simulink model "gm_sampleModel1830_1_sub_sub"  (R2023a)
settings: Solver=VariableStepAuto  StartTime=0.0  StopTime=10.0  RelTol=1e-3
libraries: hdlsllib x6, simulink x1
settings Model: Creator=user1  LastModifiedBy=user1
settings OptimizationCC: BlockReduction=off  ConditionallyExecuteInputs=off
settings DebuggingCC: InheritedTsInSrcMsg=none

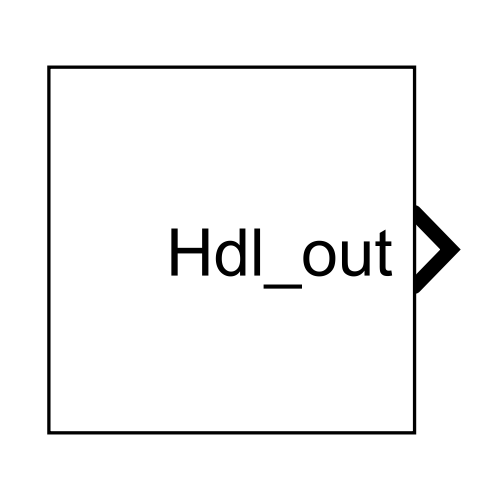
[thumbnail: Simulink's stored preview of the top-level diagram]
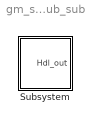
== system gm_sampleModel1830_1_sub_sub ==
  Subsystem : Subsystem

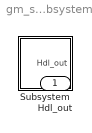
== system gm_sampleModel1830_1_sub_sub/Subsystem ==
  Subsystem : Subsystem
  Hdl_out : Outport  OutDataTypeStr=uint8

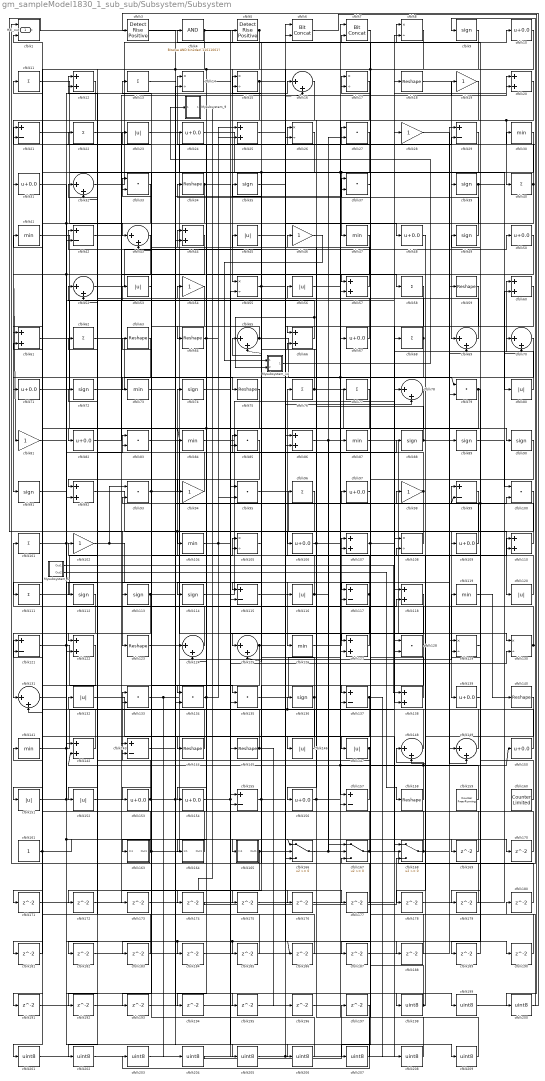
== system gm_sampleModel1830_1_sub_sub/Subsystem/Subsystem ==
  Mysubsystem_14 : Subsystem  TreatAsAtomicUnit=on  RTWFcnName=Mysubsystem_14
      settings: RTWFcnNameOpts=User specified  RTWFileNameOpts=Use function name
  Mysubsystem_5 : Subsystem  TreatAsAtomicUnit=on  RTWFcnName=Mysubsystem_5
      settings: RTWFcnNameOpts=User specified  RTWFileNameOpts=Use function name
  Mysubsystem_9 : Subsystem  TreatAsAtomicUnit=on  RTWFcnName=Mysubsystem_9
      settings: RTWFcnNameOpts=User specified  RTWFileNameOpts=Use function name
  cfblk1 : RelationalOperator  Operator=<=  OutDataTypeStr=boolean  InputSameDT=off
  cfblk{10,24,31,48,50,67,71,82,97,106,109,139,150,153..154,156} (16 alike) : Bias  Bias=0.0  SaturateOnIntegerOverflow=off
  cfblk{27,33,37,79,83,85,93,95,100,128,133..135} (13 alike) : DotProduct  OutDataTypeStr=uint8
  cfblk{11,13,22,40,58,62,68,76..77,96,101,111} (12 alike) : Sum  Inputs=+  OutDataTypeStr=uint8
  cfblk{19,28,46,54,81,94,98,102} (8 alike) : Gain  OutDataTypeStr=uint8
  cfblk{30,41,47,73,84,87,104,119,126,141} (10 alike) : MinMax  OutDataTypeStr=uint8
  cfblk{8,14..15,17,26,55,105,108,129..130} (10 alike) : Product  Inputs=*/  OutDataTypeStr=uint8  RndMeth=Zero  SaturateOnIntegerOverflow=on
  cfblk{12,20,25,44,57,60..61,66,86,92,107,110,118,122,127,138,142} (17 alike) : Sum  OutDataTypeStr=uint8
  cfblk{9,35,39,49,72,74,88..91,112..114,136} (14 alike) : Signum
  cfblk{21,29,42,99,115,117,121,137,143,155,157} (11 alike) : Sum  Inputs=+-  OutDataTypeStr=uint8
  cfblk{23,45,53,56,80,116,120,132,146..147,151..152} (12 alike) : Abs  OutDataTypeStr=uint8  SaturateOnIntegerOverflow=off
  cfblk{18,34,59,63..64,75,123,140,144..145,158} (11 alike) : Reshape
  cfblk{16,32,43,52,65,69..70,78,124..125,131,148..149} (13 alike) : Sum  Inputs=|++  OutDataTypeStr=uint8
  cfblk159 : hdlsllib/Sources/Counter Free-Running  NumBits=16  tsamp=-1
  cfblk160 : hdlsllib/Sources/Counter Limited  uplimit=7  tsamp=-1
  cfblk161 : Constant  OutDataTypeStr=uint8  SampleTime=-1
  cfblk163 : Subsystem
      settings: LibrarySourceBlock=|
      | hdlsllib/Ports &
      | Subsystems/Subsystem
  cfblk164 : Subsystem
      settings: LibrarySourceBlock=|
      | hdlsllib/Ports &
      | Subsystems/Subsystem
  cfblk165 : Subsystem
      settings: LibrarySourceBlock=|
      | hdlsllib/Ports &
      | Subsystems/Subsystem
  cfblk166 : Switch  OutDataTypeStr=uint8  SaturateOnIntegerOverflow=off  InputSameDT=off
  cfblk167 : Switch  OutDataTypeStr=uint8  SaturateOnIntegerOverflow=off  InputSameDT=off
  cfblk168 : Switch  OutDataTypeStr=uint8  SaturateOnIntegerOverflow=off  InputSameDT=off
  cfblk{169..197} (29 alike) : Delay  SampleTime=1
  cfblk{198..209} (12 alike) : DataTypeConversion  OutDataTypeStr=uint8  SaturateOnIntegerOverflow=off  RndMeth=Floor
  cfblk3 : hdlsllib/Logic and Bit Operations/Detect Rise Positive  vinit=0  OutDataTypeStr=uint8
  cfblk4 : simulink/Logic and Bit Operations/Bitwise Operator  logicop=AND  UseBitMask=on  BitMask=bin2dec('11011001')  BitMaskRealWorld=Stored Integer
      settings: LibrarySourceBlock=|
      | hdlsllib/Logic and Bit
      | Operations/Bitwise
      | Operator
  cfblk5 : hdlsllib/Logic and Bit Operations/Detect Rise Positive  vinit=0  OutDataTypeStr=uint8
  cfblk6 : hdlsllib/Logic and Bit Operations/Bit Concat  numInputs=2
  cfblk7 : hdlsllib/Logic and Bit Operations/Bit Concat  numInputs=2
  Hdl_out : Outport  OutDataTypeStr=uint8
  wires:
  cfblk11/1 -> cfblk43/1
  cfblk133/1 -> cfblk204/1, cfblk26/1
  cfblk80/1 -> cfblk60/1
  cfblk112/1 -> cfblk131/1
  cfblk120/1 -> cfblk76/1
  cfblk72/1 -> cfblk75/1
  cfblk99/1 -> cfblk139/1
  cfblk32/1 -> cfblk10/1
  cfblk10/1 -> cfblk55/1
  cfblk157/1 -> cfblk133/1
  cfblk164/1(Out1) -> cfblk102/1
  cfblk137/1 -> cfblk208/1, cfblk171/1
  cfblk52/1 -> cfblk50/1
  cfblk136/1 -> cfblk174/1, cfblk42/1
  cfblk158/1 -> cfblk142/2, cfblk148/1
  cfblk83/1 -> cfblk149/1
  cfblk1/1 -> cfblk123/1
  cfblk16/1 -> cfblk92/1
  cfblk128/1 -> cfblk175/1, cfblk52/2
  cfblk163/1(Out1) -> cfblk41/1, cfblk193/1, cfblk119/1
  cfblk98/1 -> cfblk83/1, cfblk122/1, cfblk104/1
  cfblk70/1 -> cfblk144/1
  cfblk108/1 -> cfblk106/1
  cfblk49/1 -> cfblk34/1
  cfblk18/1 -> cfblk69/1
  cfblk146/1 -> cfblk5/1
  cfblk64/1 -> cfblk25/2, cfblk84/1, cfblk134/1
  cfblk40/1 -> cfblk202/1, cfblk14/1
  cfblk30/1 -> cfblk61/1, cfblk47/1
  cfblk54/1 -> cfblk153/1
  cfblk13/1 -> cfblk205/1
  cfblk167/1 -> cfblk62/1, cfblk9/1
  cfblk75/1 -> cfblk82/1
  cfblk67/1 -> cfblk15/1
  cfblk126/1 -> cfblk107/1
  cfblk69/1 -> cfblk32/1
  cfblk37/1 -> cfblk147/1
  cfblk106/1 -> cfblk110/2, cfblk56/1
  cfblk23/1 -> cfblk145/1
  cfblk156/1 -> cfblk46/1, cfblk99/1, cfblk150/1
  cfblk119/1 -> cfblk140/1
  cfblk88/1 -> cfblk66/2, cfblk149/2
  cfblk160/1 -> cfblk99/2, cfblk4/1
  cfblk87/1 -> cfblk130/1
  cfblk20/1 -> cfblk66/1, cfblk40/1
  cfblk15/1 -> cfblk188/1, cfblk91/1
  cfblk95/1 -> cfblk120/1
  cfblk21/1 -> cfblk80/1
  cfblk142/1 -> cfblk121/1
  cfblk115/1 -> cfblk126/1
  cfblk29/1 -> cfblk73/1
  cfblk31/1 -> cfblk184/1, cfblk186/1, cfblk185/1
  cfblk41/1 -> cfblk90/1
  cfblk114/1 -> cfblk70/1
  cfblk53/1 -> cfblk33/1
  cfblk135/1 -> cfblk87/1
  cfblk90/1 -> cfblk117/1
  cfblk113/1 -> cfblk181/1, cfblk37/1
  cfblk27/1 -> cfblk37/2, cfblk33/2
  cfblk86/1 -> cfblk167/1, cfblk128/2
  cfblk148/1 -> cfblk72/1, cfblk136/1
  cfblk9/1 -> cfblk94/1, cfblk152/1
  cfblk61/1 -> cfblk143/1
  cfblk92/1 -> cfblk109/1
  cfblk116/1 -> cfblk167/2, cfblk35/1
  cfblk144/1 -> cfblk132/1
  cfblk8/1 -> cfblk166/3, cfblk57/1
  cfblk129/1 -> cfblk49/1
  cfblk58/1 -> cfblk156/1
  cfblk89/1 -> cfblk100/1
  cfblk45/1 -> cfblk48/1
  cfblk143/1 -> cfblk165/1(In1)
  cfblk12/1 -> cfblk31/1
  cfblk24/1 -> cfblk89/1
  cfblk82/1 -> cfblk20/1
  cfblk63/1 -> cfblk151/1
  cfblk74/1 -> cfblk127/1
  cfblk93/1 -> cfblk127/2, cfblk23/1
  cfblk117/1 -> cfblk93/2, cfblk146/1
  cfblk111/1 -> cfblk74/1
  cfblk168/1 -> cfblk44/1, cfblk29/1
  cfblk28/1 -> cfblk59/1
  cfblk57/1 -> cfblk21/1
  cfblk123/1 -> cfblk105/1
  cfblk59/1 -> cfblk138/2
  cfblk150/1 -> cfblk45/1
  cfblk151/1 -> cfblk16/1, cfblk209/1, cfblk166/1
  cfblk134/1 -> cfblk95/2, cfblk164/1(In1)
  cfblk4/1 -> cfblk39/1, cfblk44/2, cfblk111/1
  cfblk73/1 -> cfblk19/1
  cfblk60/1 -> cfblk86/2
  cfblk47/1 -> cfblk114/1
  cfblk34/1 -> cfblk169/1, cfblk42/2, cfblk71/1
  cfblk165/1(Out1) -> cfblk182/1, cfblk110/1
  cfblk39/1 -> cfblk70/2, cfblk154/1
  cfblk161/1 -> cfblk141/1, cfblk166/2
  cfblk166/1 -> cfblk27/2, cfblk67/1
  cfblk138/1 -> cfblk17/1
  cfblk147/1 -> cfblk107/2, cfblk143/2
  cfblk121/1 -> cfblk29/2, cfblk135/1
  cfblk65/1 -> cfblk64/1, cfblk157/1
  cfblk109/1 -> cfblk43/2
  cfblk132/1 -> cfblk168/2
  cfblk118/1 -> cfblk155/2
  cfblk44/1 -> cfblk92/2
  cfblk140/1 -> cfblk148/2
  cfblk130/1 -> cfblk61/2, cfblk30/1
  cfblk104/1 -> cfblk25/1, cfblk88/1
  cfblk100/1 -> cfblk115/1
  cfblk76/1 -> cfblk54/1, cfblk108/1
  cfblk78/1 -> cfblk137/1
  cfblk35/1 -> cfblk8/1
  cfblk159/1 -> cfblk17/2
  cfblk141/1 -> cfblk83/2, cfblk28/1
  cfblk66/1 -> cfblk52/1, Mysubsystem_14/2(In2)
  cfblk17/1 -> cfblk57/2
  cfblk26/1 -> cfblk125/1, cfblk124/2
  cfblk3/1 -> cfblk198/1
  cfblk55/1 -> cfblk170/1, cfblk125/2
  cfblk79/1 -> cfblk189/1, cfblk113/1
  cfblk125/1 -> cfblk163/1(In1), cfblk78/2
  cfblk91/1 -> cfblk115/2
  cfblk110/1 -> cfblk15/2
  cfblk94/1 -> cfblk22/1
  cfblk71/1 -> cfblk18/1
  cfblk14/1 -> cfblk116/1
  cfblk101/1 -> cfblk53/1, cfblk142/1
  cfblk145/1 -> cfblk196/1, cfblk11/1
  cfblk155/1 -> cfblk100/2, cfblk65/2
  cfblk19/1 -> cfblk134/2
  cfblk131/1 -> cfblk118/2
  cfblk22/1 -> cfblk58/1
  cfblk62/1 -> cfblk95/1
  cfblk149/1 -> cfblk24/1
  cfblk84/1 -> cfblk20/2
  cfblk85/1 -> cfblk112/1
  cfblk56/1 -> cfblk79/1, cfblk77/1
  cfblk97/1 -> cfblk27/1
  cfblk124/1 -> cfblk101/1
  cfblk105/1 -> cfblk85/1
  cfblk43/1 -> cfblk122/2, cfblk81/1
  cfblk153/1 -> cfblk12/1, cfblk199/1, cfblk98/1
  cfblk50/1 -> cfblk137/2
  cfblk68/1 -> cfblk183/1, cfblk12/2
  cfblk127/1 -> cfblk63/1
  cfblk107/1 -> cfblk187/1, cfblk68/1
  cfblk154/1 -> cfblk206/1, cfblk130/2
  cfblk102/1 -> cfblk93/1, cfblk129/1
  cfblk169/1 -> cfblk65/1
  cfblk170/1 -> cfblk133/2
  cfblk171/1 -> cfblk124/1
  cfblk96/1 -> cfblk172/1
  cfblk172/1 -> cfblk78/1
  cfblk42/1 -> cfblk173/1
  cfblk173/1 -> cfblk155/1
  cfblk174/1 -> cfblk168/3
  cfblk175/1 -> cfblk168/1
  cfblk152/1 -> cfblk176/1
  cfblk176/1 -> cfblk8/2
  cfblk177/1 -> cfblk1/2
  cfblk48/1 -> cfblk178/1
  cfblk178/1 -> cfblk60/2
  cfblk139/1 -> cfblk179/1
  cfblk179/1 -> cfblk1/1
  cfblk180/1 -> cfblk105/2
  cfblk181/1 -> cfblk121/2
  cfblk182/1 -> cfblk69/2
  cfblk183/1 -> cfblk32/2
  cfblk184/1 -> cfblk86/1
  cfblk185/1 -> cfblk131/2
  cfblk186/1 -> cfblk21/2
  cfblk187/1 -> cfblk79/2
  cfblk188/1 -> cfblk167/3
  cfblk189/1 -> cfblk129/2
  cfblk25/1 -> cfblk190/1
  cfblk190/1 -> cfblk118/1
  cfblk122/1 -> cfblk191/1
  cfblk191/1 -> cfblk26/2
  cfblk33/1 -> cfblk192/1
  cfblk192/1 -> cfblk14/2
  cfblk193/1 -> cfblk135/2
  cfblk5/1 -> Hdl_out/1, cfblk194/1
  cfblk194/1 -> cfblk55/2
  cfblk81/1 -> cfblk195/1
  cfblk195/1 -> cfblk117/2
  cfblk196/1 -> cfblk157/2
  cfblk198/1 -> cfblk108/2, cfblk97/1
  cfblk199/1 -> cfblk3/1
  cfblk6/1 -> cfblk200/1
  cfblk200/1 -> cfblk180/1
  cfblk77/1 -> cfblk201/1
  cfblk201/1 -> cfblk6/1
  cfblk202/1 -> cfblk6/2
  cfblk197/1 -> cfblk203/1
  cfblk203/1 -> cfblk85/2
  cfblk204/1 -> cfblk197/1
  cfblk205/1 -> cfblk128/1, cfblk16/2
  cfblk206/1 -> cfblk13/1
  cfblk7/1 -> cfblk207/1
  cfblk207/1 -> cfblk96/1
  cfblk208/1 -> cfblk7/1
  cfblk209/1 -> cfblk7/2
  Mysubsystem_5/1(Out1) -> cfblk138/1
  Mysubsystem_5/2(Out2) -> cfblk158/1
  Mysubsystem_9/1(Out1) -> cfblk177/1
  cfblk46/1 -> Mysubsystem_14/1(In1)
  Mysubsystem_14/1(Out1) -> Mysubsystem_9/1(In1)

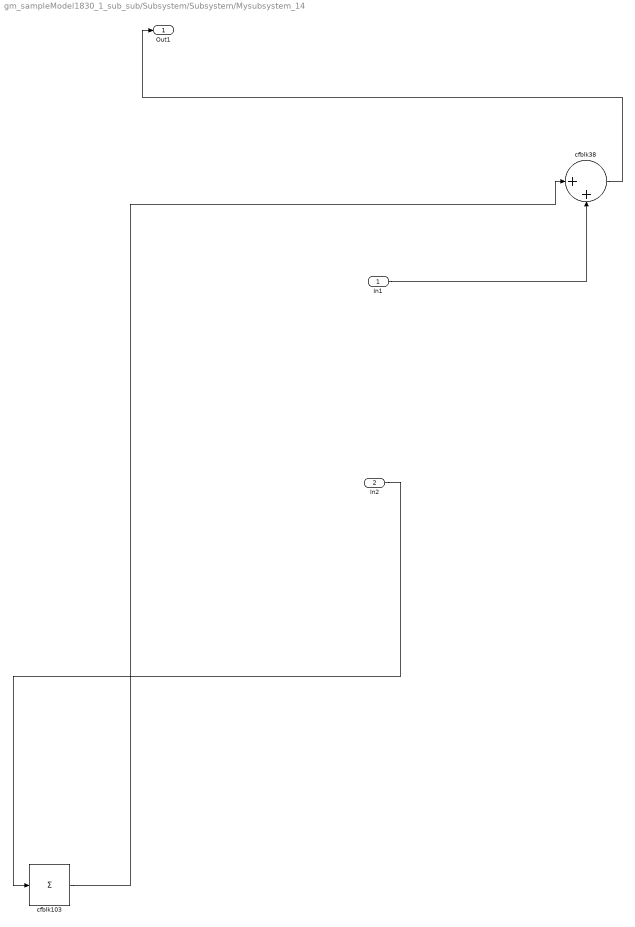
== system gm_sampleModel1830_1_sub_sub/Subsystem/Subsystem/Mysubsystem_14 ==
  In1 : Inport
  In2 : Inport  Port=2
  cfblk103 : Sum  Inputs=+
  cfblk38 : Sum  Inputs=|++
  Out1 : Outport
  wires:
  In2/1 -> cfblk103/1
  In1/1 -> cfblk38/2
  cfblk103/1 -> cfblk38/1
  cfblk38/1 -> Out1/1

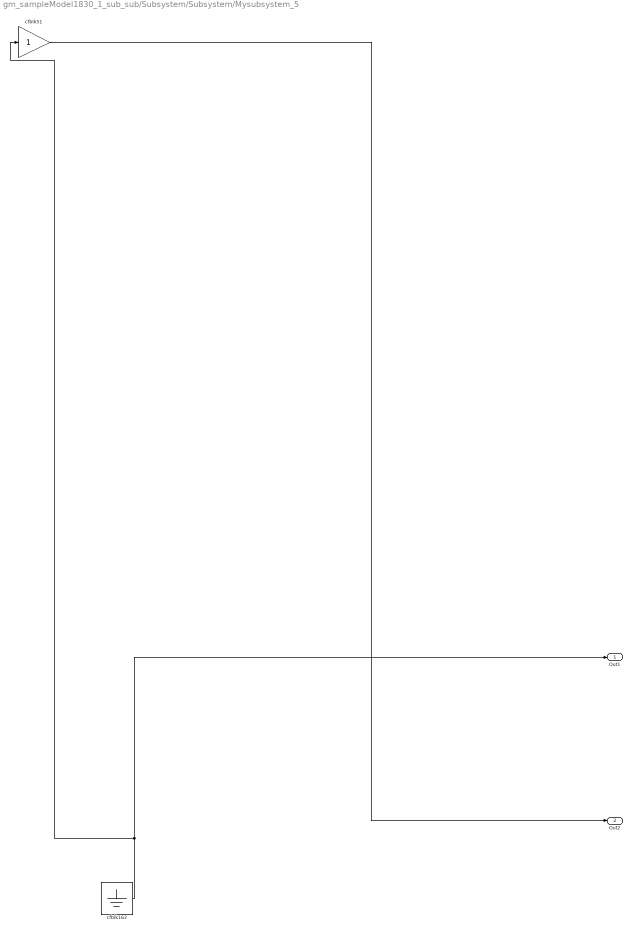
== system gm_sampleModel1830_1_sub_sub/Subsystem/Subsystem/Mysubsystem_5 ==
  cfblk162 : Ground
  cfblk51 : Gain
  Out1 : Outport
  Out2 : Outport  Port=2
  wires:
  cfblk51/1 -> Out2/1
  cfblk162/1 -> cfblk51/1, Out1/1

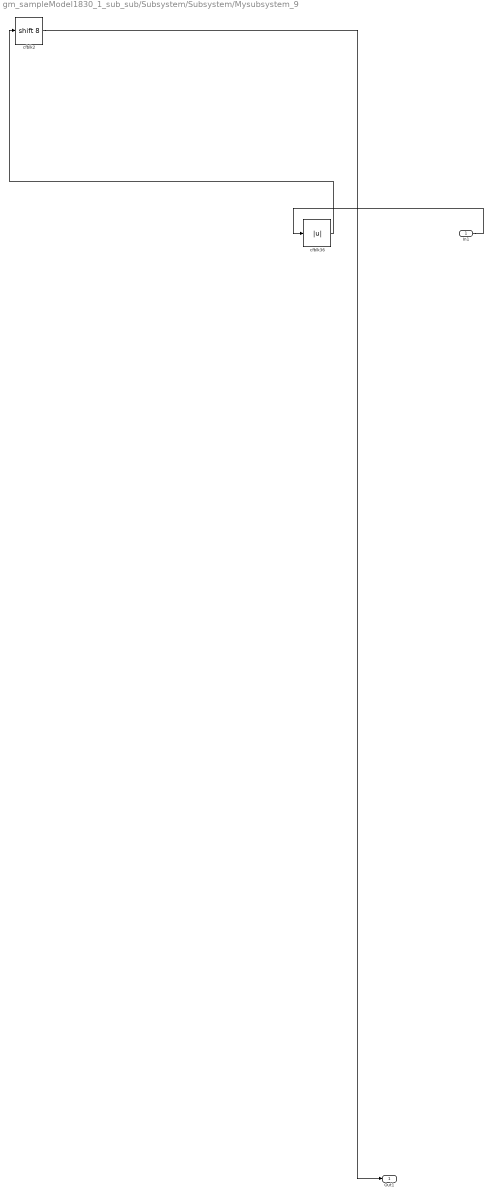
== system gm_sampleModel1830_1_sub_sub/Subsystem/Subsystem/Mysubsystem_9 ==
  In1 : Inport
  cfblk2 : ArithShift  BitShiftNumber=8
  cfblk36 : Abs  SaturateOnIntegerOverflow=off
  Out1 : Outport
  wires:
  In1/1 -> cfblk36/1
  cfblk2/1 -> Out1/1
  cfblk36/1 -> cfblk2/1

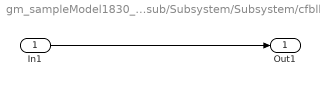
== system gm_sampleModel1830_1_sub_sub/Subsystem/Subsystem/cfblk163 ==
  In1 : Inport
  Out1 : Outport
  wires:
  In1/1 -> Out1/1

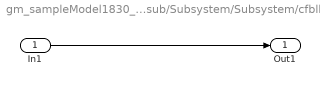
== system gm_sampleModel1830_1_sub_sub/Subsystem/Subsystem/cfblk164 ==
  In1 : Inport
  Out1 : Outport
  wires:
  In1/1 -> Out1/1

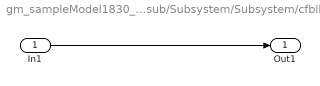
== system gm_sampleModel1830_1_sub_sub/Subsystem/Subsystem/cfblk165 ==
  In1 : Inport
  Out1 : Outport
  wires:
  In1/1 -> Out1/1
